simulink model "design"  (R2019b)
settings: Solver=FixedStepAuto  StartTime=0.0  StopTime=40  FixedStep=0.01  RelTol=1e-3
values from neighbouring files (symbols this model uses):
  A = [0 0 1 0 0 0 0.0009 0 0 ... (first row only)    [H2_design.m]    (also in H2_design.mat = [0 0 0 0 0 0 0 0 0 0 0 0 ... (81 elements, 9x9)])
  Acmp = A+B*F+K*C1    [H2_design.m]    (also in H2_design.mat = [-1.24023079432 -0.00155492056242 -1637.55791223 -0.02523616)
  B = [0 0 0 ... (first row only)    [H2_design.m]    (also in H2_design.mat = [0 0 0 0 0.2026 2.5878 0 0 0 0 0 0 ... (27 elements, 9x3)])
  Bcmp = -K    [H2_design.m]    (also in H2_design.mat = [1.24023079432 0.00155492056242 0.325539221186 0.02523616035)
  C1 = [1 0 0 0 0 0 0 0 0 ... (first row only)    [H2_design.m]    (also in H2_design.mat = [1 0 0 0 0 0 0 1 0 0 0 0 ... (54 elements, 6x9)])
  C2 = [1 0 0 0 0 0 0 0 0 ... (first row only)    [H2_design.m]    (also in H2_design.mat = [1 0 0 0 1 0 0 0 0 0 0 0 ... (27 elements, 3x9)])
  Ccmp = F    [H2_design.m]    (also in H2_design.mat = [-92.5170676293 4.00955631135 -37.7560015453 -2.815079291 -9)
  D1 = zeros(6,3)    [H2_design.m]    (also in H2_design.mat = [0 0 0 0 0 0 0 0 0 0 0 0 ... (18 elements, 6x3)])
  E = [0 0 0 ... (first row only)    [H2_design.m]    (also in H2_design.mat = [0 0 -0.0001 0 0 0 -0.002 0 0 0 0 0.1756 ... (27 elements, 9)
  x0 = [0 -0.1 0 0 0 0 0 0 0.1]'    [H2_design.m]    (also in H2_design.mat = [0 -0.1 0 0 0 0 0 0 0.1])
settings Model: Creator=allen  LastModifiedBy=allen

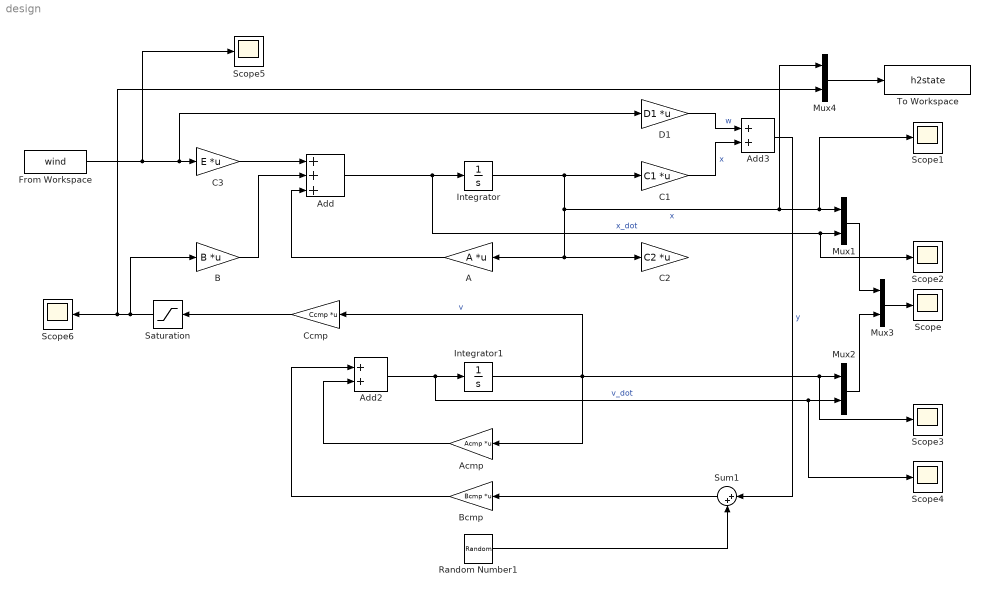
== system design ==
  A : Gain  Gain=A  Multiplication=Matrix(K*u)
  Acmp : Gain  Gain=Acmp  Multiplication=Matrix(K*u)
  Add : Sum  Inputs=+++
  Add2 : Sum
  Add3 : Sum
  B : Gain  Gain=B  Multiplication=Matrix(K*u)
  Bcmp : Gain  Gain=Bcmp  Multiplication=Matrix(K*u)
  C1 : Gain  Gain=C1  Multiplication=Matrix(K*u)
  C2 : Gain  Gain=C2  Multiplication=Matrix(K*u)
  C3 : Gain  Gain=E  Multiplication=Matrix(K*u)
  Ccmp : Gain  Gain=Ccmp  Multiplication=Matrix(K*u)
  D1 : Gain  Gain=D1  Multiplication=Matrix(K*u)
  From Workspace : FromWorkspace  VariableName=wind  SampleTime=0
  Integrator : Integrator  InitialCondition=x0
  Integrator1 : Integrator
  Mux{1..4} (4 alike) : Mux  Inputs=2
  Random Number1 : RandomNumber  Variance=0.01  Seed=10  SampleTime=0.1
  Saturation : Saturate  UpperLimit=[0.35;0.35;0.4]  LowerLimit=[-0.35;-0.35;-0.4]
  Scope{,1..6} (7 alike) : Scope
  Sum1 : Sum  Inputs=|++
  To Workspace : ToWorkspace  VariableName=h2state  SampleTime=-1
  wires:
  Add/1 -> Scope2/1, Mux1/2, Integrator/1  "x_dot"
  Integrator/1 -> C2/1, A/1, Mux4/1, Scope1/1, Mux1/1, C1/1  "x"
  A/1 -> Add/3
  C3/1 -> Add/1
  B/1 -> Add/2
  Acmp/1 -> Add2/2
  Bcmp/1 -> Add2/1
  Add2/1 -> Scope4/1, Mux2/2, Integrator1/1  "v_dot"
  Integrator1/1 -> Ccmp/1, Scope3/1, Mux2/1, Acmp/1  "v"
  D1/1 -> Add3/1  "w"
  C1/1 -> Add3/2  "x"
  Mux1/1 -> Mux3/1
  Mux2/1 -> Mux3/2
  Mux3/1 -> Scope/1
  From Workspace/1 -> Scope5/1, D1/1, C3/1
  Saturation/1 -> Mux4/2, Scope6/1, B/1
  Ccmp/1 -> Saturation/1
  Add3/1 -> Sum1/1  "y"
  Sum1/1 -> Bcmp/1
  Random Number1/1 -> Sum1/2
  Mux4/1 -> To Workspace/1
